simulink library "Encoder"  (Simulink 8.0)
settings: Solver=ode45  StartTime=0.0  StopTime=10.0  RelTol=1e-3
libraries: simulink x7
settings Model: Creator=Juliano  LastModifiedBy=h3now

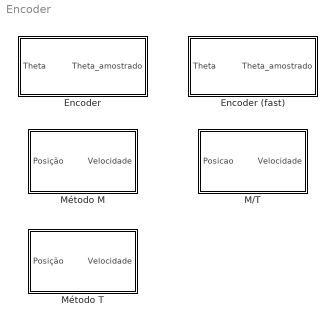
== system Encoder ==
  Encoder : Subsystem  mask(Encoder de quadratura){Nr=360}
      mask prompts: Nr "Número de pulsos por revolução"
      mask help:
      | Simula o funcionamento de um encoder de quadratura.
      |
      | Entradas
      | - Theta: ângulo real [graus]
      | Saídas
      | - Theta_amostrado: ângulo que um encoder mostraria [graus]
  Encoder (fast) : Subsystem  mask(Encoder de quadratura (fast)){Nr=360}
      mask help:
      | Simula o funcionamento de um encoder de quadratura sem ter de simular cada um dos pulsos gerados pelos sensores ópticos.
      |
      | ATENÇÃO: NÃO DEVE SER UTILIZADO PARA ALIMENTAR NEM O MÉTODO T NEM O MÉTODO M/T PARA CÁLCULO DE VELOCIDADE.
      |
      | Entradas
      | - Theta: ângulo real [graus]
      | Saídas
      | - Theta_amostrado: ângulo que um encoder mostraria [graus]
  M/T : Subsystem  mask{Ts=0.1}
      mask prompts: Ts "Sampling time"
      mask help:
      | Calcula a velocidade por meio do método M/T de medição: Conta o número de pulsos durante Ts segundos (onde Ts é o tempo pré-determinado pelo usuário + tempo necessário para contar um número inteiro de pulsos).
      |
      | Entradas
      | -Posição: Essa entrada deve ser conectada à saída do bloco "Encoder" dessa biblioteca.
      | Saída
      | -Velocidade: Estimativa da velocidade dada pelo método M/T [graus/s]
  Método M : Subsystem  mask(Método de medição de velocidade M){Ts=0.1}
      mask prompts: Ts "Tempo de amostragem [s]"
      mask help:
      | Calcula a velocidade por meio do método M de medição: Conta pulsos durante um tempo pré-determinado e calcula a velocidade média.
      |
      | Entradas
      | -Posição: Essa entrada deve ser conectada à saída do bloco "Encoder" dessa biblioteca.
      | Saída
      | -Velocidade: Estimativa da velocidade dada pelo método M [graus/s]
  Método T : Subsystem  mask(Método de medição de velocidade T){m=1}
      mask prompts: m "Número de pulsos que o bloco espera para calcular a velocidade média"
      mask help:
      | Calcula a velocidade por meio do método T de medição: Conta o tempo durante um número pré-determinado de pulsos e calcula a velocidade média.
      |
      | Entradas
      | -Posição: Essa entrada deve ser conectada à saída do bloco "Encoder" dessa biblioteca.
      | Saída
      | -Velocidade: Estimativa da velocidade dada pelo método M [graus/s]

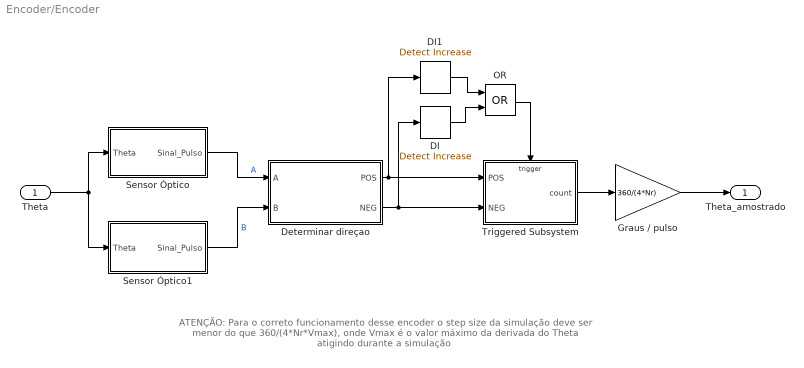
== system Encoder/Encoder ==
  note: ATENÇÃO: Para o correto funcionamento desse encoder o step size da simulação deve ser menor do que 360/(4*Nr*Vmax),
      | onde Vmax é o valor máximo da derivada do Theta atigindo durante a simulação
  Theta : Inport
  DI : simulink/Logic and Bit Operations/Detect Increase  vinit=0.0  InputProcessing=Inherited  OutDataTypeStr=boolean
  DI1 : simulink/Logic and Bit Operations/Detect Increase  vinit=0.0  InputProcessing=Inherited  OutDataTypeStr=boolean
  Determinar direçao : Subsystem
  Graus / pulso : Gain  Gain=360/(4*Nr)  OutDataTypeStr=double
  OR : Logic  Operator=OR  AllPortsSameDT=off  OutDataTypeStr=boolean
  Sensor Óptico : Subsystem
  Sensor Óptico1 : Subsystem
  Triggered Subsystem : Subsystem  TreatAsAtomicUnit=on
  Theta_amostrado : Outport
  wires:
  Sensor Óptico/1(Sinal_Pulso) -> Determinar direçao/1(A)  "A"
  Sensor Óptico1/1(Sinal_Pulso) -> Determinar direçao/2(B)  "B"
  Triggered Subsystem/1(count) -> Graus / pulso/1
  Graus / pulso/1 -> Theta_amostrado/1
  Theta/1 -> Sensor Óptico1/1(Theta), Sensor Óptico/1(Theta)
  Determinar direçao/1(POS) -> DI1/1, Triggered Subsystem/1(POS)
  Determinar direçao/2(NEG) -> Triggered Subsystem/2(NEG), DI/1
  DI1/1 -> OR/1
  DI/1 -> OR/2
  OR/1 -> Triggered Subsystem/Trigger

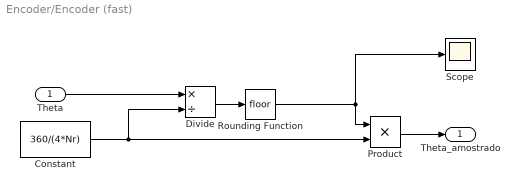
== system Encoder/Encoder (fast) ==
  "Theta " : Inport
  Constant : Constant  Value=360/(4*Nr)
  Divide : Product  Inputs=*/
  Product : Product  RndMeth=Zero
  Rounding Function : Rounding
  Scope : Scope
  Theta_amostrado : Outport
  wires:
  Divide/1 -> Rounding Function/1
  Rounding Function/1 -> Scope/1, Product/1
  "Theta "/1 -> Divide/1
  Constant/1 -> Product/2, Divide/2
  Product/1 -> Theta_amostrado/1

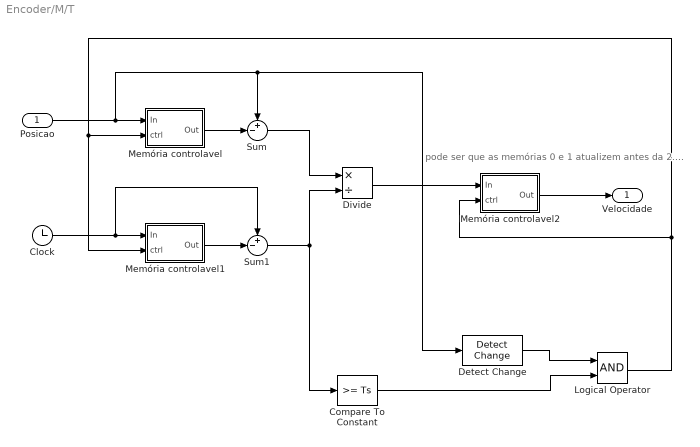
== system Encoder/M/T ==
  note: pode ser que as memórias 0 e 1 atualizem antes da 2....
  Posicao : Inport
  Clock : Clock
  Compare To Constant : simulink/Logic and Bit Operations/Compare To Constant  relop=>=  const=Ts  OutDataTypeStr=boolean
  Detect Change : simulink/Logic and Bit Operations/Detect Change  vinit=0  InputProcessing=Inherited  OutDataTypeStr=boolean
  Divide : Product  Inputs=*/
  Logical Operator : Logic  AllPortsSameDT=off  OutDataTypeStr=boolean
  Memória controlavel : Subsystem
  Memória controlavel1 : Subsystem
  Memória controlavel2 : Subsystem
  Sum : Sum  Inputs=+-|
  Sum1 : Sum  Inputs=+-|
  Velocidade : Outport
  wires:
  Posicao/1 -> Detect Change/1, Sum/1, Memória controlavel/1(In)
  Sum1/1 -> Compare To Constant/1, Divide/2
  Memória controlavel/1(Out) -> Sum/2
  Divide/1 -> Memória controlavel2/1(In)
  Clock/1 -> Memória controlavel1/1(In), Sum1/1
  Memória controlavel1/1(Out) -> Sum1/2
  Sum/1 -> Divide/1
  Compare To Constant/1 -> Logical Operator/2
  Detect Change/1 -> Logical Operator/1
  Logical Operator/1 -> Memória controlavel1/2(ctrl), Memória controlavel/2(ctrl), Memória controlavel2/2(ctrl)
  Memória controlavel2/1(Out) -> Velocidade/1

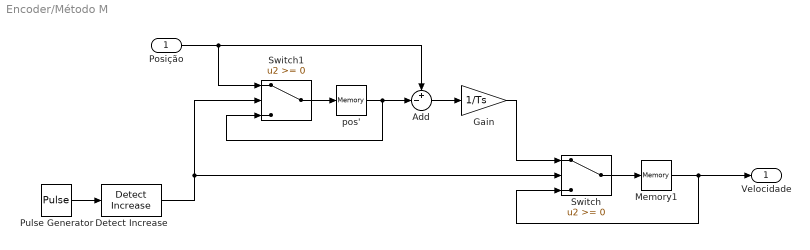
== system Encoder/Método M ==
  Posição : Inport
  Add : Sum  Inputs=+-|
  Detect Increase : simulink/Logic and Bit Operations/Detect Increase  vinit=0.0  InputProcessing=Inherited  OutDataTypeStr=boolean
  Gain : Gain  Gain=1/Ts
  Memory1 : Memory
  Pulse Generator : DiscretePulseGenerator  PulseType=Time based  Period=Ts  PulseWidth=50
  Switch : Switch
  Switch1 : Switch
  pos' : Memory
  Velocidade : Outport
  wires:
  pos'/1 -> Add/2, Switch1/3
  Pulse Generator/1 -> Detect Increase/1
  Add/1 -> Gain/1
  Switch1/1 -> pos'/1
  Switch/1 -> Memory1/1
  Memory1/1 -> Velocidade/1, Switch/3
  Posição/1 -> Switch1/1, Add/1
  Gain/1 -> Switch/1
  Detect Increase/1 -> Switch/2, Switch1/2

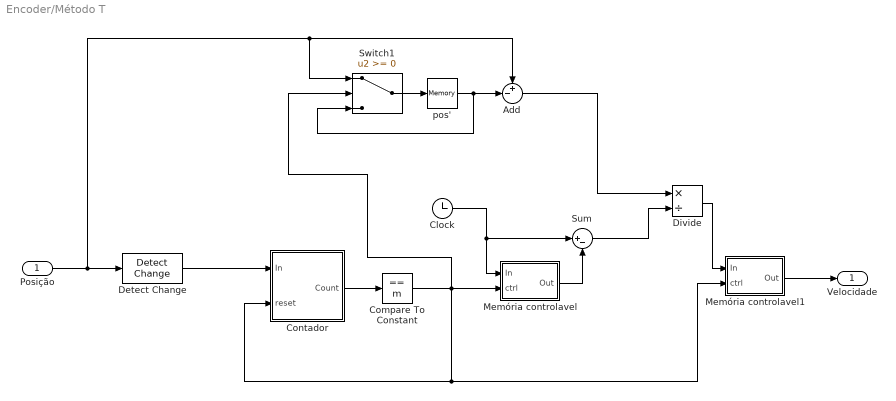
== system Encoder/Método T ==
  Posição : Inport
  Add : Sum  Inputs=+-|
  Clock : Clock
  Compare To Constant : simulink/Logic and Bit Operations/Compare To Constant  relop===  const=m  OutDataTypeStr=boolean
  Contador : Subsystem
  Detect Change : simulink/Logic and Bit Operations/Detect Change  vinit=0  InputProcessing=Inherited  OutDataTypeStr=boolean
  Divide : Product  Inputs=*/
  Memória controlavel : Subsystem
  Memória controlavel1 : Subsystem
  Sum : Sum  Inputs=|+-
  Switch1 : Switch
  pos' : Memory
  Velocidade : Outport
  wires:
  Posição/1 -> Switch1/1, Add/1, Detect Change/1
  Detect Change/1 -> Contador/1(In)
  Contador/1(Count) -> Compare To Constant/1
  Divide/1 -> Memória controlavel1/1(In)
  Memória controlavel/1(Out) -> Sum/2
  Sum/1 -> Divide/2
  Add/1 -> Divide/1
  Clock/1 -> Sum/1, Memória controlavel/1(In)
  Compare To Constant/1 -> Memória controlavel1/2(ctrl), Contador/2(reset), Switch1/2, Memória controlavel/2(ctrl)
  Memória controlavel1/1(Out) -> Velocidade/1
  pos'/1 -> Add/2, Switch1/3
  Switch1/1 -> pos'/1

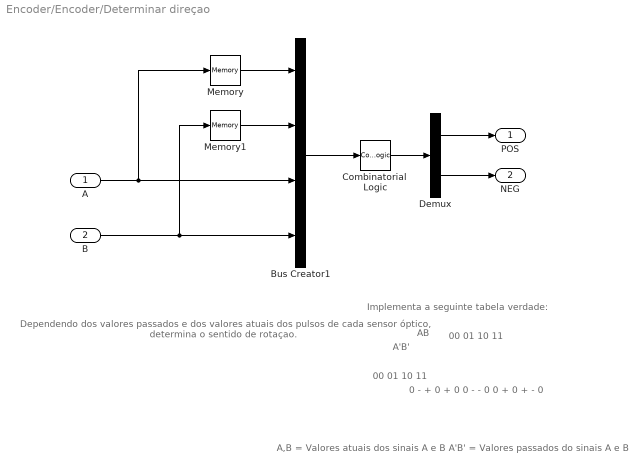
== system Encoder/Encoder/Determinar direçao ==
  note: A,B = Valores atuais dos sinais A e B
      | A'B' = Valores passados do sinais A e B
  note: A'B'
  note: AB
  note: Implementa a seguinte tabela verdade:
  note: 0	-	+	0
      | +	0	0	-
      | -	0	0	+
      | 0	+	-	0
  note: 00 01 10 11
  note: 00
      | 01
      | 10
      | 11
  note: Dependendo dos valores passados e dos valores atuais
      | dos pulsos de cada sensor óptico, determina o sentido
      | de rotaçao.
  A : Inport
  B : Inport  Port=2
  Bus Creator1 : BusCreator
  Combinatorial  Logic : CombinatorialLogic  TruthTable=[ 0 0 ; 0 1 ; 1 0 ; 0 0 ; 1 0 ; 0 0 ; 0 0 ; 0 1 ; 0 1 ; 0 0 ; 0 0 ; 1 0 ; 0 0 ; 1 0 ; 0 1 ; 0 0]
  Demux : Demux  Outputs=2
  Memory : Memory
  Memory1 : Memory
  POS : Outport
  NEG : Outport  Port=2
  wires:
  Demux/1 -> POS/1
  A/1 -> Memory/1, Bus Creator1/3
  Demux/2 -> NEG/1
  Combinatorial  Logic/1 -> Demux/1
  Memory/1 -> Bus Creator1/1
  Bus Creator1/1 -> Combinatorial  Logic/1
  Memory1/1 -> Bus Creator1/2
  B/1 -> Memory1/1, Bus Creator1/4

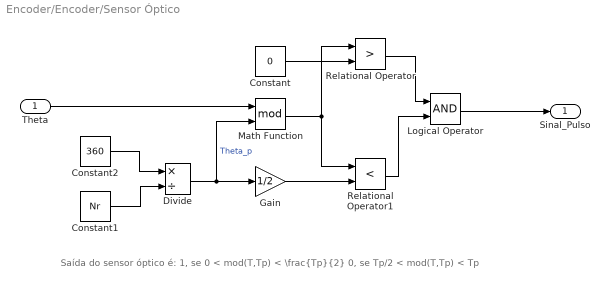
== system Encoder/Encoder/Sensor Óptico ==
  note: Saída do sensor óptico é:
      | 1, se	0 < mod(T,Tp) < \frac{Tp}{2}
      |  0, se      Tp/2 < mod(T,Tp) < Tp
  Theta : Inport
  Constant : Constant  Value=0
  Constant1 : Constant  Value=Nr
  Constant2 : Constant  Value=360
  Divide : Product  Inputs=*/
  Gain : Gain  Gain=1/2
  Logical Operator : Logic  AllPortsSameDT=off  OutDataTypeStr=boolean
  Math Function : Math  Operator=mod  SaturateOnIntegerOverflow=on
  Relational Operator : RelationalOperator  Operator=>  OutDataTypeStr=boolean
  Relational Operator1 : RelationalOperator  Operator=<  OutDataTypeStr=boolean
  Sinal_Pulso : Outport
  wires:
  Math Function/1 -> Relational Operator1/1, Relational Operator/1
  Theta/1 -> Math Function/1
  Relational Operator/1 -> Logical Operator/1
  Relational Operator1/1 -> Logical Operator/2
  Constant/1 -> Relational Operator/2
  Divide/1 -> Math Function/2, Gain/1  "Theta_p"
  Gain/1 -> Relational Operator1/2
  Logical Operator/1 -> Sinal_Pulso/1
  Constant2/1 -> Divide/1
  Constant1/1 -> Divide/2

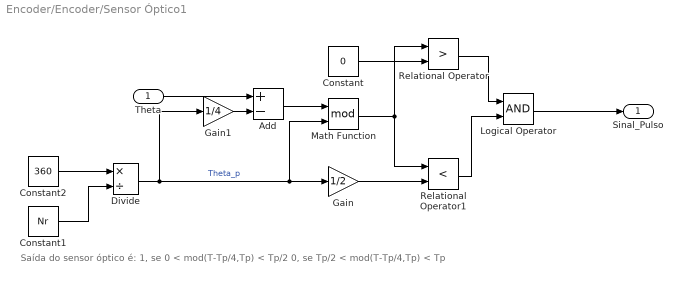
== system Encoder/Encoder/Sensor Óptico1 ==
  note: Saída do sensor óptico é:
      | 1, se	0 < mod(T-Tp/4,Tp) < Tp/2
      |  0, se     Tp/2 < mod(T-Tp/4,Tp) < Tp
  Theta : Inport
  Add : Sum  Inputs=+-
  Constant : Constant  Value=0
  Constant1 : Constant  Value=Nr
  Constant2 : Constant  Value=360
  Divide : Product  Inputs=*/
  Gain : Gain  Gain=1/2
  Gain1 : Gain  Gain=1/4
  Logical Operator : Logic  AllPortsSameDT=off  OutDataTypeStr=boolean
  Math Function : Math  Operator=mod  SaturateOnIntegerOverflow=on
  Relational Operator : RelationalOperator  Operator=>  OutDataTypeStr=boolean
  Relational Operator1 : RelationalOperator  Operator=<  OutDataTypeStr=boolean
  Sinal_Pulso : Outport
  wires:
  Constant1/1 -> Divide/2
  Constant2/1 -> Divide/1
  Logical Operator/1 -> Sinal_Pulso/1
  Gain/1 -> Relational Operator1/2
  Divide/1 -> Gain1/1, Gain/1, Math Function/2  "Theta_p"
  Constant/1 -> Relational Operator/2
  Relational Operator1/1 -> Logical Operator/2
  Relational Operator/1 -> Logical Operator/1
  Math Function/1 -> Relational Operator/1, Relational Operator1/1
  Add/1 -> Math Function/1
  Theta/1 -> Add/1
  Gain1/1 -> Add/2

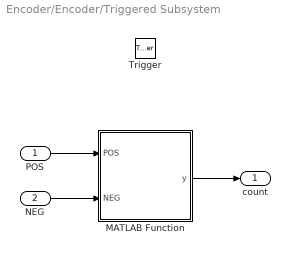
== system Encoder/Encoder/Triggered Subsystem ==
  POS : Inport
  NEG : Inport  Port=2
  Trigger : TriggerPort
  MATLAB Function : MATLAB Function  TreatAsAtomicUnit=on
  count : Outport
  wires:
  POS/1 -> MATLAB Function/1(POS)
  NEG/1 -> MATLAB Function/2(NEG)
  MATLAB Function/1(y) -> count/1

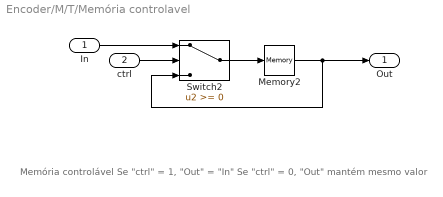
== system Encoder/M/T/Memória controlavel ==
  note: Memória controlável
      |
      | Se "ctrl" = 1, "Out" = "In"
      | Se "ctrl" = 0, "Out" mantém mesmo valor
  In : Inport
  ctrl : Inport  Port=2
  Memory2 : Memory
  Switch2 : Switch
  Out : Outport
  wires:
  In/1 -> Switch2/1
  ctrl/1 -> Switch2/2
  Memory2/1 -> Switch2/3, Out/1
  Switch2/1 -> Memory2/1

== system Encoder/M/T/Memória controlavel1 ==
  note: Memória controlável
      |
      | Se "ctrl" = 1, "Out" = "In"
      | Se "ctrl" = 0, "Out" mantém mesmo valor
  In : Inport
  ctrl : Inport  Port=2
  Memory2 : Memory
  Switch2 : Switch
  Out : Outport
  wires:
  Switch2/1 -> Memory2/1
  Memory2/1 -> Out/1, Switch2/3
  ctrl/1 -> Switch2/2
  In/1 -> Switch2/1

== system Encoder/M/T/Memória controlavel2 ==
  note: Memória controlável
      |
      | Se "ctrl" = 1, "Out" = "In"
      | Se "ctrl" = 0, "Out" mantém mesmo valor
  In : Inport
  ctrl : Inport  Port=2
  Memory2 : Memory
  Switch2 : Switch
  Out : Outport
  wires:
  Switch2/1 -> Memory2/1
  Memory2/1 -> Out/1, Switch2/3
  ctrl/1 -> Switch2/2
  In/1 -> Switch2/1

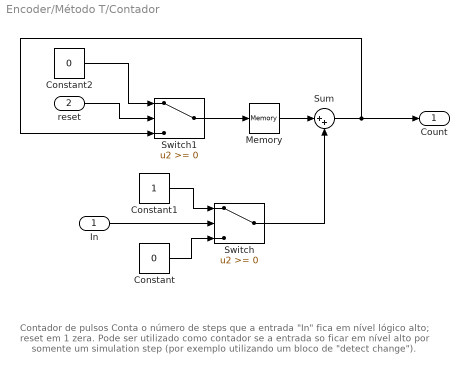
== system Encoder/Método T/Contador ==
  note: Contador de pulsos
      |
      | Conta o número de steps que a entrada "In" fica em nível lógico alto; reset em 1 zera.
      | Pode ser utilizado como contador se a entrada so ficar em nível alto por somente um
      | simulation step (por exemplo utilizando um bloco de "detect change").
  In : Inport
  reset : Inport  Port=2
  Constant : Constant  Value=0
  Constant1 : Constant
  Constant2 : Constant  Value=0
  Memory : Memory
  Sum : Sum  Inputs=|++
  Switch : Switch
  Switch1 : Switch
  Count : Outport
  wires:
  Switch1/1 -> Memory/1
  Constant2/1 -> Switch1/1
  reset/1 -> Switch1/2
  In/1 -> Switch/2
  Switch/1 -> Sum/2
  Sum/1 -> Count/1, Switch1/3
  Constant1/1 -> Switch/1
  Memory/1 -> Sum/1
  Constant/1 -> Switch/3

== system Encoder/Método T/Memória controlavel ==
  note: Memória controlável
      |
      | Se "ctrl" = 1, "Out" = "In"
      | Se "ctrl" = 0, "Out" mantém mesmo valor
  In : Inport
  ctrl : Inport  Port=2
  Memory2 : Memory
  Switch2 : Switch
  Out : Outport
  wires:
  Switch2/1 -> Memory2/1
  Memory2/1 -> Out/1, Switch2/3
  ctrl/1 -> Switch2/2
  In/1 -> Switch2/1

== system Encoder/Método T/Memória controlavel1 ==
  note: Memória controlável
      |
      | Se "ctrl" = 1, "Out" = "In"
      | Se "ctrl" = 0, "Out" mantém mesmo valor
  In : Inport
  ctrl : Inport  Port=2
  Memory2 : Memory
  Switch2 : Switch
  Out : Outport
  wires:
  In/1 -> Switch2/1
  ctrl/1 -> Switch2/2
  Memory2/1 -> Switch2/3, Out/1
  Switch2/1 -> Memory2/1

== matlab function Encoder/Triggered Subsystem/MATLAB Function ==
  data: POS input double; y output double; NEG input double
function y = fcn(POS,NEG)
%#codegen
persistent count;
persistent last_update;

if(isempty(count))
    count = -1;
    last_update = 1;
end

if(POS==1)&&(last_update==1)||(NEG==1)&&(last_update==-1)
    if(POS==1)
        count = count +1;
        last_update = 1;
    elseif(NEG==1)
        count = count -1;
        last_update = -1;
    end
elseif(POS==1)
    last_update = 1;
elseif(NEG==1)
    last_update = -1;
end


y = count;
